simulink model "DC_Motor_Response_Check"  (R2016b)
settings: Solver=FixedStepAuto  StartTime=0.0  StopTime=10.0  RelTol=1e-3  EnableMultiTasking=on
libraries: RASPlib x3, MinSegLibrary_M2V3 x2
settings Model: ExtModeTrigDuration=2  Creator=Sang  LastModifiedBy=Sang
settings OptimizationCC: MaxStackSize=64
settings DebuggingCC: ParameterTunabilityLossMsg=error
settings HardwareCC: ProdBitPerInt=16  ProdBitPerPointer=16  ProdBitPerSizeT=16  ProdBitPerPtrDiffT=16  ProdLargestAtomicFloat=None  ProdWordSize=8  ProdHWDeviceType=Atmel->AVR
settings RTWCC: SystemTargetFile=ert.tlc  HardwareBoard=Arduino Mega 2560  TLCOptions=-aInlineSetEventsForThisBaseRateFcn=TLC_FALSE -aSuppressMultiTaskScheduler=TLC_FALSE -aRateBasedStepFcn=1  TemplateMakefile=ert_default_tmf  Description=Embedded Coder  GenerateReport=on  Toolchain=Arduino AVR  BuildConfiguration=Faster Runs  IncludeHyperlinkInReport=on  LaunchReport=on  GenerateTraceInfo=on  GenerateTraceReport=on  GenerateTraceReportSl=on  GenerateTraceReportSf=on  GenerateTraceReportEml=on
settings CodeAppCC: ForceParamTrailComments=on  IgnoreCustomStorageClasses=off  OperatorAnnotations=on  SimulinkDataObjDesc=on  SFDataObjDesc=on  MATLABFcnDesc=on  InsertBlockDesc=on  MATLABSourceComments=on
settings ERTTargetCC: SupportContinuousTime=on  SupportVariableSizeSignals=on

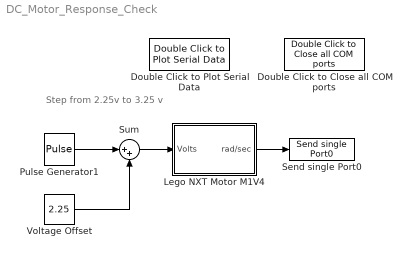
== system DC_Motor_Response_Check ==
  note: Step from 2.25v
      | to 3.25 v
  Double Click to Close all COM ports : RASPlib/Double Click to Close all COM ports
  Double Click to Plot Serial Data : RASPlib/Double Click to Plot Serial Data  COMport=4  BaudRate=9600  NumSamples=500  DataType=single
  Lego NXT Motor M1V4 : Subsystem
  Pulse Generator1 : DiscretePulseGenerator  PulseType=Time based  Period=9  PulseWidth=50
  Send single Port0 : RASPlib/Send single Port0
  Sum : Sum  Inputs=|++
  Voltage Offset : Constant  Value=2.25
  wires:
  Lego NXT Motor M1V4/1(rad/sec) -> Send single Port0/1
  Pulse Generator1/1 -> Sum/1
  Voltage Offset/1 -> Sum/2
  Sum/1 -> Lego NXT Motor M1V4/1(Volts)

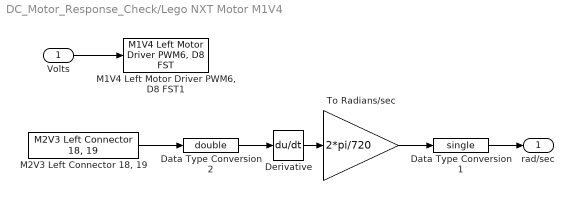
== system DC_Motor_Response_Check/Lego NXT Motor M1V4 ==
  Volts : Inport
  Data Type Conversion1 : DataTypeConversion  OutDataTypeStr=single
  Data Type Conversion2 : DataTypeConversion  OutDataTypeStr=double
  Derivative : Derivative
  "M1V4 Left Motor Driver PWM6, D8 FST1" : MinSegLibrary_M2V3/M1V4 Left Motor Driver PWM6, D8 FST  Vsupply=3.25
  "M2V3 Left Connector 18, 19" : MinSegLibrary_M2V3/M2V3 Left Connector 18, 19  Encoder=1  PinA=19  PinB=18  PWMFSelect=3  PWMTimer=-1
  To Radians/sec : Gain  Gain=2*pi/720
  rad/sec : Outport
  wires:
  Derivative/1 -> To Radians/sec/1
  Volts/1 -> "M1V4 Left Motor Driver PWM6, D8 FST1"/1
  To Radians/sec/1 -> Data Type Conversion1/1
  "M2V3 Left Connector 18, 19"/1 -> Data Type Conversion2/1
  Data Type Conversion2/1 -> Derivative/1
  Data Type Conversion1/1 -> rad/sec/1
